simulink model "ex_3"  (R2023a)
settings: Solver=FixedStepAuto  StartTime=0.0  StopTime=100  FixedStep=1e-4  RelTol=1e-3
settings Model: Creator=LabCom  LastModifiedBy=LabCom

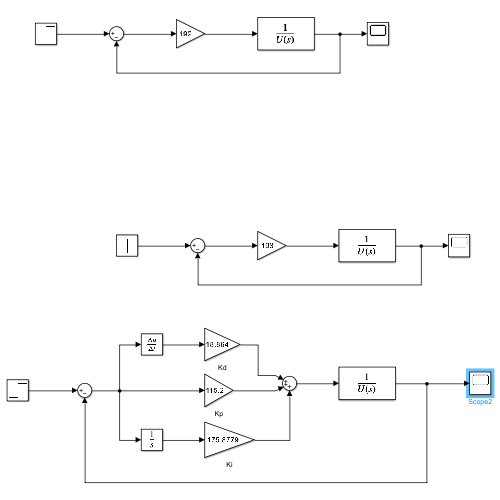
[thumbnail: Simulink's stored preview of the top-level diagram]
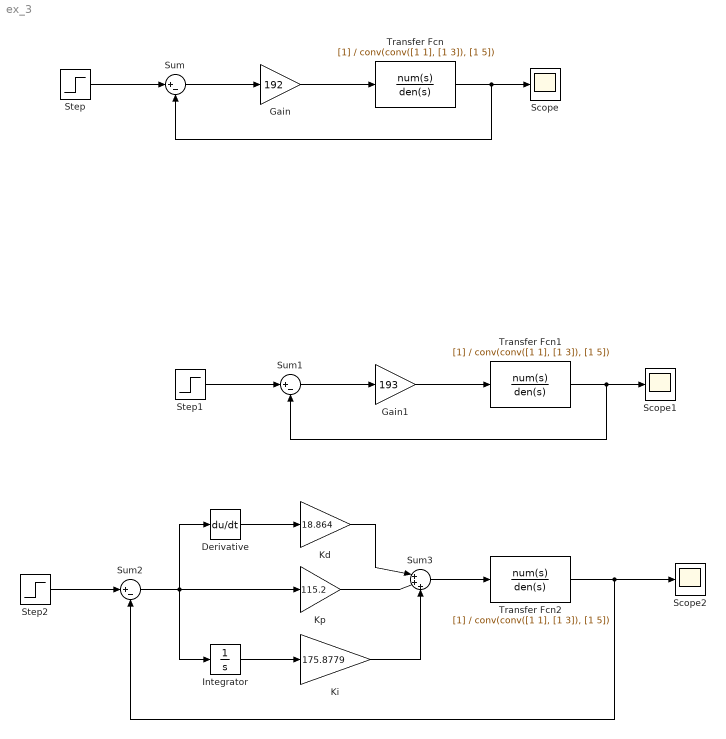
== system ex_3 ==
  Derivative : Derivative
  Gain : Gain  Gain=192
  Gain1 : Gain  Gain=193
  Integrator : Integrator
  Kd : Gain  Gain=18.864
  Ki : Gain  Gain=175.8779
  Kp : Gain  Gain=115.2
  Scope : Scope
  Scope1 : Scope
  Scope2 : Scope
  Step : Step  Time=0  SampleTime=0
  Step1 : Step  Time=0  SampleTime=0
  Step2 : Step  Time=0  SampleTime=0
  Sum : Sum  Inputs=|+-
  Sum1 : Sum  Inputs=|+-
  Sum2 : Sum  Inputs=|+-
  Sum3 : Sum  Inputs=|+++
  Transfer Fcn : TransferFcn  Denominator=conv(conv([1 1], [1 3]), [1 5])
  Transfer Fcn1 : TransferFcn  Denominator=conv(conv([1 1], [1 3]), [1 5])
  Transfer Fcn2 : TransferFcn  Denominator=conv(conv([1 1], [1 3]), [1 5])
  wires:
  Step/1 -> Sum/1
  Sum/1 -> Gain/1
  Transfer Fcn/1 -> Sum/2, Scope/1
  Gain/1 -> Transfer Fcn/1
  Transfer Fcn1/1 -> Sum1/2, Scope1/1
  Sum1/1 -> Gain1/1
  Gain1/1 -> Transfer Fcn1/1
  Step1/1 -> Sum1/1
  Ki/1 -> Sum3/3
  Transfer Fcn2/1 -> Scope2/1, Sum2/2
  Sum3/1 -> Transfer Fcn2/1
  Kd/1 -> Sum3/1
  Integrator/1 -> Ki/1
  Derivative/1 -> Kd/1
  Kp/1 -> Sum3/2
  Step2/1 -> Sum2/1
  Sum2/1 -> Derivative/1, Integrator/1, Kp/1
